simulink model "simulator_prototype_v2"  (R2021b)
settings: Solver=VariableStepAuto  StartTime=0.0  StopTime=60  FixedStep=0.0001  RelTol=1e-4
values from neighbouring files (symbols this model uses):
  N = length(mass)    [inertia_matrix.m]
undefined symbols (not defined in the file or in its folder): X, Y, Z
libraries: sm_lib x47, nesl_utility x7
(part 3 of 12)

== matlab function simulator_prototype_v2/Dynamic Model/MATLAB Function ==
  data: b input; D_q output; dq input
function D_q = dissipative_vector(b, dq)
    D_q = zeros(6,1);
    for i = 1:6
        D_q(i) = b*dq(i);
    end
end
